simulink model "Full_Project"  (R2019b)
settings: Solver=ode5  StartTime=0.0  StopTime=inf  FixedStep=0.05  RelTol=1e-3  EnableMultiTasking=on
libraries: arduinolib x3
settings Model: SILPILModeSetting=veronly  ExtModeTrigDuration=2  Creator=semir  LastModifiedBy=semir
settings SolverCC: AutoInsertRateTranBlk=on
settings OptimizationCC: EnhancedBackFolding=on  PassReuseOutputArgsAs=Individual arguments  ZeroExternalMemoryAtStartup=off  ZeroInternalMemoryAtStartup=off  MaxStackSize=64  OptimizeBlockOrder=speed  DifferentSizesBufferReuse=on  OptimizationCustomize=off  EfficientTunableParamExpr=on
settings DebuggingCC: ParameterTunabilityLossMsg=error
settings HardwareCC: ProdBitPerInt=16  ProdBitPerPointer=16  ProdBitPerSizeT=16  ProdBitPerPtrDiffT=16  ProdLargestAtomicFloat=None  ProdWordSize=8  ProdHWDeviceType=Atmel->AVR  UseEmbeddedCoderFeatures=off  UseSimulinkCoderFeatures=off
settings SFSimCC: MATLABDynamicMemAlloc=off
settings RTWCC: SystemTargetFile=ert.tlc  HardwareBoard=Arduino Uno  TLCOptions=-aInlineSetEventsForThisBaseRateFcn=TLC_FALSE -aSuppressMultiTaskScheduler=TLC_FALSE -aRateBasedStepFcn=1  TemplateMakefile=ert_default_tmf  GenerateReport=on  Toolchain=Arduino AVR  BuildConfiguration=Faster Runs  IncludeHyperlinkInReport=on  LaunchReport=on  GenerateTraceInfo=on  GenerateTraceReport=on  GenerateTraceReportSl=on  GenerateTraceReportSf=on  GenerateTraceReportEml=on
settings CodeAppCC: ForceParamTrailComments=on  IgnoreCustomStorageClasses=off  OperatorAnnotations=on  SimulinkDataObjDesc=on  SFDataObjDesc=on  InsertBlockDesc=on
settings ERTTargetCC: SupportContinuousTime=on  SupportNonInlinedSFcns=on  SupportVariableSizeSignals=on  ExtModeStaticAllocSize=250

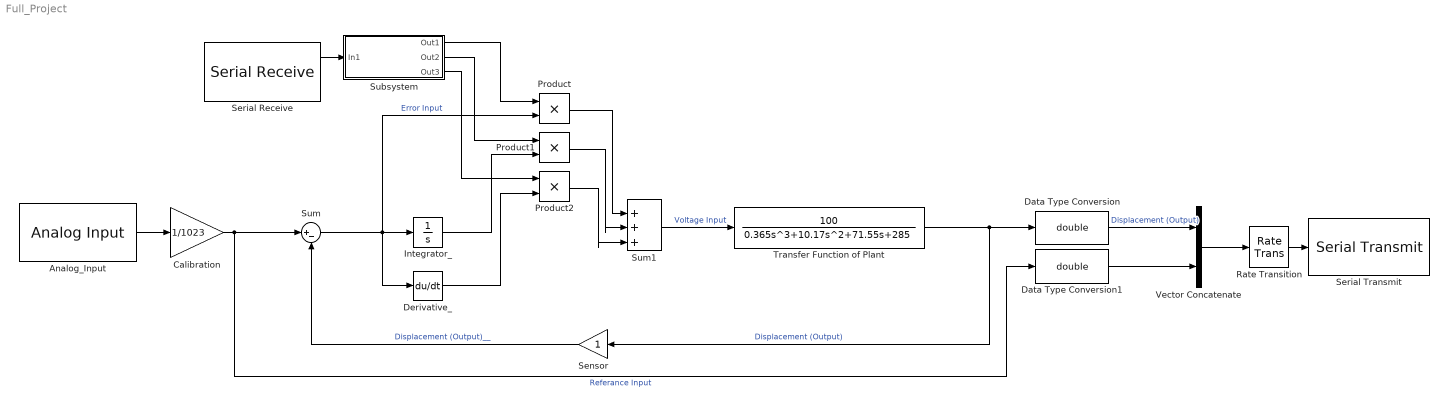
== system Full_Project ==
  Analog_Input : arduinolib/Analog Input  pinNumber=4  ReadResultsOnly=off  ConversionTriggerSource=Software  ExternalTriggerType=uint32(0)  OutputDataType=uint16  EnableConversionCompleteNotify=off  EnableOuputStatus=off  SampleTime=-1  blockPlatform=arduino
  Calibration : Gain  Gain=1/1023
  Data Type Conversion : DataTypeConversion  OutDataTypeStr=double
  Data Type Conversion1 : DataTypeConversion  OutDataTypeStr=double
  Derivative_ : Derivative
  Integrator_ : Integrator
  Product : Product
  Product1 : Product
  Product2 : Product
  Rate Transition : RateTransition  OutPortSampleTime=0.1
  Sensor : Gain
  Serial Receive : arduinolib/Serial Receive  isARMArch=off  portNumber=0  DataType=int8  Datalength=8  SampleTime=0.05  showOutStatus=on  blockPlatform=arduino
      settings: SourceProductName=Simulink Support Package for Arduino Hardware  SourceProductBaseCode=ARDUINO
  Serial Transmit : arduinolib/Serial Transmit  portNumber=0  sendmode=println  sendformat=Decimal  floatprecision=2  blockPlatform=arduino
      settings: SourceProductName=Simulink Support Package for Arduino Hardware
  Subsystem : Subsystem
  Sum : Sum  Inputs=|+-
  Sum1 : Sum  Inputs=|+++
  Transfer Function of Plant : TransferFcn  Numerator=[100]  Denominator=[0.365 10.17 71.55 285]
  Vector Concatenate : Concatenate
  wires:
  Product1/1 -> Sum1/2
  Derivative_/1 -> Product2/2
  Product/1 -> Sum1/1
  Subsystem/3(Out3) -> Product2/1
  Product2/1 -> Sum1/3
  Subsystem/1(Out1) -> Product/1
  Integrator_/1 -> Product1/2
  Subsystem/2(Out2) -> Product1/1
  Calibration/1 -> Data Type Conversion1/1, Sum/1  "Referance Input"
  Sum/1 -> Product/2, Derivative_/1, Integrator_/1  "Error Input"
  Sensor/1 -> Sum/2  "Displacement (Output)__"
  Analog_Input/1 -> Calibration/1
  Sum1/1 -> Transfer Function of Plant/1  "Voltage Input"
  Transfer Function of Plant/1 -> Sensor/1, Data Type Conversion/1  "Displacement (Output)"
  Vector Concatenate/1 -> Rate Transition/1
  Rate Transition/1 -> Serial Transmit/1
  Data Type Conversion/1 -> Vector Concatenate/1  "Displacement (Output)"
  Data Type Conversion1/1 -> Vector Concatenate/2
  Serial Receive/1 -> Subsystem/1(In1)

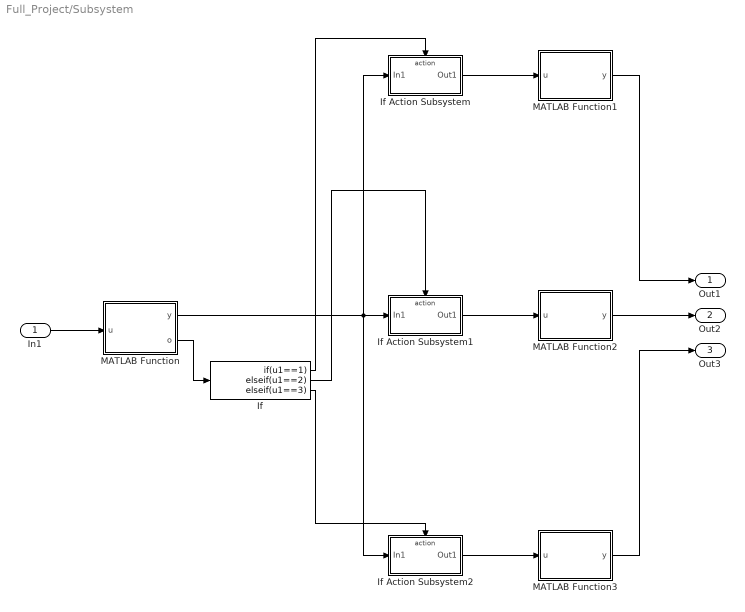
== system Full_Project/Subsystem ==
  In1 : Inport
  If : If  IfExpression=u1==1  ElseIfExpressions=u1==2,u1==3  ShowElse=off
  If Action Subsystem : Subsystem  TreatAsAtomicUnit=on
  If Action Subsystem1 : Subsystem  TreatAsAtomicUnit=on
  If Action Subsystem2 : Subsystem  TreatAsAtomicUnit=on
  MATLAB Function : MATLAB Function  TreatAsAtomicUnit=on
  MATLAB Function1 : MATLAB Function  TreatAsAtomicUnit=on
  MATLAB Function2 : MATLAB Function  TreatAsAtomicUnit=on
  MATLAB Function3 : MATLAB Function  TreatAsAtomicUnit=on
  Out1 : Outport
  Out2 : Outport  Port=2
  Out3 : Outport  Port=3
  wires:
  If Action Subsystem1/1(Out1) -> MATLAB Function2/1(u)
  MATLAB Function3/1(y) -> Out3/1
  MATLAB Function/1(y) -> If Action Subsystem2/1(In1), If Action Subsystem/1(In1), If Action Subsystem1/1(In1)
  If Action Subsystem2/1(Out1) -> MATLAB Function3/1(u)
  If Action Subsystem/1(Out1) -> MATLAB Function1/1(u)
  MATLAB Function1/1(y) -> Out1/1
  If/1 -> If Action Subsystem/Action
  If/3 -> If Action Subsystem2/Action
  MATLAB Function/2(o) -> If/1
  If/2 -> If Action Subsystem1/Action
  MATLAB Function2/1(y) -> Out2/1
  In1/1 -> MATLAB Function/1(u)

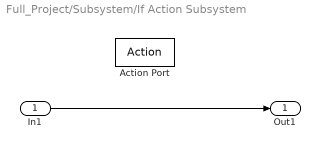
== system Full_Project/Subsystem/If Action Subsystem ==
  In1 : Inport
  Action Port : ActionPort  ActionPortLabel=if(u1==1)
  Out1 : Outport
  wires:
  In1/1 -> Out1/1

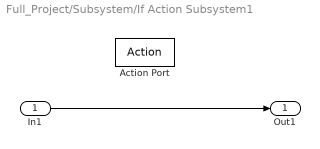
== system Full_Project/Subsystem/If Action Subsystem1 ==
  In1 : Inport
  Action Port : ActionPort  ActionPortLabel=elseif(u1==2)
  Out1 : Outport
  wires:
  In1/1 -> Out1/1

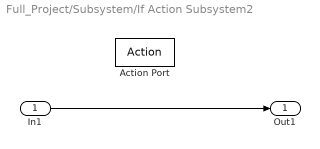
== system Full_Project/Subsystem/If Action Subsystem2 ==
  In1 : Inport
  Action Port : ActionPort  ActionPortLabel=elseif(u1==3)
  Out1 : Outport
  wires:
  In1/1 -> Out1/1

== matlab function Full_Project/Subsystem/MATLAB Function ==
  data: u input; y output; o output
function [y,o]= fcn(u)
    % k==>107 p==>112 i==>105 d==>100
    o=0;
    if u(8)==112
        o=1;
    elseif u(8)==105
        o=2;
    elseif u(8)==100
        o=3;
    end
    y=u;
end

== matlab function Full_Project/Subsystem/MATLAB Function1 ==
  data: u input; y output
function y = fcn(u)
    r1 = Switcher(u(1));   % Arduino üzerinden gelen 8 bitlik bilginin 1.bitinin Switcher fonksiyonunda kullanılması
    r2 = Switcher(u(2));   % Arduino üzerinden gelen 8 bitlik bilginin 2.bitinin Switcher fonksiyonunda kullanılması
    r3 = Switcher(u(3));   % Arduino üzerinden gelen 8 bitlik bilginin 3.bitinin Switcher fonksiyonunda kullanılması
    r4 = Switcher(u(4));   % Arduino üzerinden gelen 8 bitlik bilginin 4.bitinin Switcher fonksiyonunda kullanılması
    r5 = Switcher(u(5));   % Arduino üzerinden gelen 8 bitlik bilginin 5.bitinin Switcher fonksiyonunda kullanılması
    r6 = Switcher(u(6));   % Arduino üzerinden gelen 8 bitlik bilginin 6.bitinin Switcher fonksiyonunda kullanılması
    r7 = Switcher(u(7));   % Arduino üzerinden gelen 8 bitlik bilginin 7.bitinin Switcher fonksiyonunda kullanılması
    r8 = Switcher(u(8));   % Arduino üzerinden gelen 8 bitlik bilginin 8.bitinin Switcher fonksiyonunda kullanılması
    y = (r1)*10^(2)+(r2)*10^(1)+(r3)*10^(0)+(r4)*10^(0)+(r5)*10^(-1)+(r6)*10^(-2)+(r7)*10^(0)+(r8)*10^(0);
end

% Gelen ASCII kodunun rakam olup olmamasına göre ayrıştırılma fonksiyonu
function result = Switcher(in)
    switch in
        case 48
            result = 0;
        case 49
            result = 1;
        case 50
            result = 2;
        case 51
            result = 3;
        case 52
            result = 4;
        case 53
            result = 5;
        case 54
            result = 6;
        case 55
            result = 7;
        case 56
            result = 8;
        case 57
            result = 9;
        otherwise
            result = 0;
    end
end

== matlab function Full_Project/Subsystem/MATLAB Function2 ==
  data: u input; y output
function y = fcn(u)
    r1 = Switcher(u(1));   % Arduino üzerinden gelen 8 bitlik bilginin 1.bitinin Switcher fonksiyonunda kullanılması
    r2 = Switcher(u(2));   % Arduino üzerinden gelen 8 bitlik bilginin 2.bitinin Switcher fonksiyonunda kullanılması
    r3 = Switcher(u(3));   % Arduino üzerinden gelen 8 bitlik bilginin 3.bitinin Switcher fonksiyonunda kullanılması
    r4 = Switcher(u(4));   % Arduino üzerinden gelen 8 bitlik bilginin 4.bitinin Switcher fonksiyonunda kullanılması
    r5 = Switcher(u(5));   % Arduino üzerinden gelen 8 bitlik bilginin 5.bitinin Switcher fonksiyonunda kullanılması
    r6 = Switcher(u(6));   % Arduino üzerinden gelen 8 bitlik bilginin 6.bitinin Switcher fonksiyonunda kullanılması
    r7 = Switcher(u(7));   % Arduino üzerinden gelen 8 bitlik bilginin 7.bitinin Switcher fonksiyonunda kullanılması
    r8 = Switcher(u(8));   % Arduino üzerinden gelen 8 bitlik bilginin 8.bitinin Switcher fonksiyonunda kullanılması
    y = (r1)*10^(2)+(r2)*10^(1)+(r3)*10^(0)+(r4)*10^(0)+(r5)*10^(-1)+(r6)*10^(-2)+(r7)*10^(0)+(r8)*10^(0);
end

% Gelen ASCII kodunun rakam olup olmamasına göre ayrıştırılma fonksiyonu
function result = Switcher(in)
    switch in
        case 48
            result = 0;
        case 49
            result = 1;
        case 50
            result = 2;
        case 51
            result = 3;
        case 52
            result = 4;
        case 53
            result = 5;
        case 54
            result = 6;
        case 55
            result = 7;
        case 56
            result = 8;
        case 57
            result = 9;
        otherwise
            result = 0;
    end
end

== matlab function Full_Project/Subsystem/MATLAB Function3 ==
  data: u input; y output
function y = fcn(u)
    r1 = Switcher(u(1));   % Arduino üzerinden gelen 8 bitlik bilginin 1.bitinin Switcher fonksiyonunda kullanılması
    r2 = Switcher(u(2));   % Arduino üzerinden gelen 8 bitlik bilginin 2.bitinin Switcher fonksiyonunda kullanılması
    r3 = Switcher(u(3));   % Arduino üzerinden gelen 8 bitlik bilginin 3.bitinin Switcher fonksiyonunda kullanılması
    r4 = Switcher(u(4));   % Arduino üzerinden gelen 8 bitlik bilginin 4.bitinin Switcher fonksiyonunda kullanılması
    r5 = Switcher(u(5));   % Arduino üzerinden gelen 8 bitlik bilginin 5.bitinin Switcher fonksiyonunda kullanılması
    r6 = Switcher(u(6));   % Arduino üzerinden gelen 8 bitlik bilginin 6.bitinin Switcher fonksiyonunda kullanılması
    r7 = Switcher(u(7));   % Arduino üzerinden gelen 8 bitlik bilginin 7.bitinin Switcher fonksiyonunda kullanılması
    r8 = Switcher(u(8));   % Arduino üzerinden gelen 8 bitlik bilginin 8.bitinin Switcher fonksiyonunda kullanılması
    y = (r1)*10^(2)+(r2)*10^(1)+(r3)*10^(0)+(r4)*10^(0)+(r5)*10^(-1)+(r6)*10^(-2)+(r7)*10^(0)+(r8)*10^(0);
end

% Gelen ASCII kodunun rakam olup olmamasına göre ayrıştırılma fonksiyonu
function result = Switcher(in)
    switch in
        case 48
            result = 0;
        case 49
            result = 1;
        case 50
            result = 2;
        case 51
            result = 3;
        case 52
            result = 4;
        case 53
            result = 5;
        case 54
            result = 6;
        case 55
            result = 7;
        case 56
            result = 8;
        case 57
            result = 9;
        otherwise
            result = 0;
    end
end
